simulink model "double_star_controlled_rectifier"  (Simulink 6.1)
settings: Solver=ode23tb  StartTime=0.0  StopTime=0.1499  MaxStep=5e-5  RelTol=1e-3  AbsTol=.01
libraries: powerlib x19
settings Model: LastModifiedBy=cloud
settings DebuggingCC: SolverPrmCheckMsg=warning

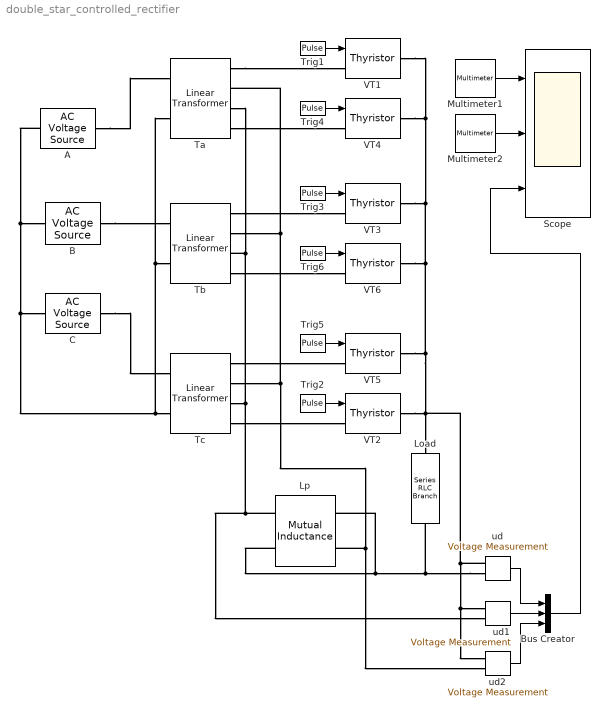
== system double_star_controlled_rectifier ==
  A : powerlib/Electrical Sources/AC Voltage Source  Amplitude=150  Phase=30  Frequency=50  SampleTime=0  Measurements=Voltage
  B : powerlib/Electrical Sources/AC Voltage Source  Amplitude=150  Phase=-90  Frequency=50  SampleTime=0  Measurements=Voltage
  Bus Creator : BusCreator  DialogController=Simulink.DDGSource_Bus  Inputs=3
  C : powerlib/Electrical Sources/AC Voltage Source  Amplitude=150  Phase=-210  Frequency=50  SampleTime=0  Measurements=Voltage
  Load : powerlib/Elements/Series RLC Branch  Orientation=down  PhysicalDomain=powersysdomain  SubClassName=unknown  LeftPortType=p1  RightPortType=p1  LConnTagsString=__new0  RConnTagsString=__new0  Resistance=5  Inductance=0.1  Capacitance=inf  Measurements=Branch voltage and current
  Lp : powerlib/Elements/Mutual Inductance  Orientation=left  PhysicalDomain=powersysdomain  SubClassName=unknown  LeftPortType=p1  RightPortType=p1  LConnTagsString=a|b  RConnTagsString=A|B  SelfImpedance1=[0.5 5.1e-02]  SelfImpedance2=[0.5 5.1e-02]  ThreeWindings=off  SelfImpedance3=[ 1.1 1.1e-03]  MutualImpedance=[0 5.0e-02]  Measurements=None
      settings: AttributesFormatString=\n
  Multimeter1 : powerlib/Measurements/Multimeter  PhasorSimulation=off  OutputType=Complex  sel=[11 12 13]  L=26  Gain=[1 1 1]  yselected={'Usrc: A','Usrc: B','Usrc: C'};  PSBOutputType=1  PSBequivalent=0  AxesSetting=[0,0.1,-100,100]  Display=0  SavedBlockNames=-11
  Multimeter2 : powerlib/Measurements/Multimeter  PhasorSimulation=off  OutputType=Complex  sel=[16 17]  L=26  Gain=[-1 1]  yselected={'Iw2: Ta','Iw3: Ta'};  PSBOutputType=1  PSBequivalent=0  AxesSetting=[0,0.1,-100,100]  Display=0  SavedBlockNames=-11
  Scope : Scope  NumInputPorts=3
      settings: TimeRange=0.05  YMin=-200~-20~-200  YMax=200~20~200  Decimation=5  SampleTime=1e-4
  Ta : powerlib/Elements/Linear Transformer  PhysicalDomain=powersysdomain  SubClassName=unknown  LeftPortType=p1  RightPortType=p1  LConnTagsString=a|b  RConnTagsString=A|B|C|D  NominalPower=[ 10000 50 ]  winding1="[ 100  0.002  0.08 ]"  winding2="[ 100  0.002  0.08 ]"  ThreeWindings=on  winding3=[ 100 0.002 0.08 ]  RmLm=[ 500 500 ]  Measurements=All voltages and currents
  Tb : powerlib/Elements/Linear Transformer  PhysicalDomain=powersysdomain  SubClassName=unknown  LeftPortType=p1  RightPortType=p1  LConnTagsString=a|b  RConnTagsString=A|B|C|D  NominalPower=[ 10000 50 ]  winding1="[ 100  0.002  0.08 ]"  winding2="[ 100  0.002  0.08 ]"  ThreeWindings=on  winding3=[ 100 0.002 0.08 ]  RmLm=[ 500 500 ]  Measurements=All voltages and currents
  Tc : powerlib/Elements/Linear Transformer  PhysicalDomain=powersysdomain  SubClassName=unknown  LeftPortType=p1  RightPortType=p1  LConnTagsString=a|b  RConnTagsString=A|B|C|D  NominalPower=[ 10000 50 ]  winding1="[ 100  0.002  0.08 ]"  winding2="[ 100  0.002  0.08 ]"  ThreeWindings=on  winding3=[ 100 0.002 0.08 ]  RmLm=[ 500 500 ]  Measurements=All voltages and currents
  Trig1 : DiscretePulseGenerator  PulseType=Time based  Amplitude=10  Period=0.02  PulseWidth=20  PhaseDelay=0.00167
  Trig2 : DiscretePulseGenerator  PulseType=Time based  Amplitude=10  Period=0.02  PulseWidth=20  PhaseDelay=0.005
  Trig3 : DiscretePulseGenerator  PulseType=Time based  Amplitude=10  Period=0.02  PulseWidth=20  PhaseDelay=0.008333
  Trig4 : DiscretePulseGenerator  PulseType=Time based  Amplitude=10  Period=0.02  PulseWidth=20  PhaseDelay=0.01167
  Trig5 : DiscretePulseGenerator  PulseType=Time based  Amplitude=10  Period=0.02  PulseWidth=20  PhaseDelay=0.015
  Trig6 : DiscretePulseGenerator  PulseType=Time based  Amplitude=10  Period=0.02  PulseWidth=20  PhaseDelay=0.01833
  VT{1..6} (6 alike) : powerlib/Power Electronics/Thyristor  Ron=0.01  Lon=0  Vf=0.8  IC=0  Rs=1000  Cs=100e-9  Measurements=off
  ud : powerlib/Measurements/Voltage Measurement  PhasorSimulation=off  OutputType=Complex  PSBequivalent=0
  ud1 : powerlib/Measurements/Voltage Measurement  PhasorSimulation=off  OutputType=Complex  PSBequivalent=0
  ud2 : powerlib/Measurements/Voltage Measurement  PhasorSimulation=off  OutputType=Complex  PSBequivalent=0
  wires:
  Trig1/1 -> VT1/1
  Trig4/1 -> VT4/1
  Trig3/1 -> VT3/1
  Trig6/1 -> VT6/1
  Trig5/1 -> VT5/1
  Trig2/1 -> VT2/1
  Multimeter1/1 -> Scope/1
  Multimeter2/1 -> Scope/2
  ud/1 -> Bus Creator/1
  ud1/1 -> Bus Creator/2
  ud2/1 -> Bus Creator/3
  Bus Creator/1 -> Scope/3
  connections:
  A/LConn1 -- B/LConn1 -- C/LConn1 -- Ta/LConn2 -- Tb/LConn2 -- Tc/LConn2
  B/RConn1 -- Tb/LConn1
  A/RConn1 -- Ta/LConn1
  Tc/RConn2 -- Ta/RConn2 -- Tb/RConn2 -- Lp/LConn2 -- ud2/LConn2
  Lp/RConn1 -- Tc/RConn3 -- Ta/RConn3 -- Tb/RConn3 -- ud1/LConn2
  Ta/RConn1 -- VT1/LConn1
  Ta/RConn4 -- VT4/LConn1
  Tb/RConn1 -- VT3/LConn1
  Tb/RConn4 -- VT6/LConn1
  Tc/RConn4 -- VT2/LConn1
  Tc/RConn1 -- VT5/LConn1
  ud/LConn2 -- Lp/RConn2 -- Lp/LConn1 -- Load/RConn1
  VT5/RConn1 -- ud2/LConn1 -- ud1/LConn1 -- ud/LConn1 -- Load/LConn1 -- VT2/RConn1 -- VT1/RConn1 -- VT4/RConn1 -- VT3/RConn1 -- VT6/RConn1
  C/RConn1 -- Tc/LConn1
